simulink model "multi_model"  (R2016b)
settings: Solver=ode15s  StartTime=0.0  StopTime=inf  FixedStep=0.001  MaxStep=0.004  RelTol=1e-3
InitFcn:
  | kR_old=0;
  | kOm_old=0;
undefined symbols (not defined in the file): deg, rad, s
libraries: simulink x23, aerolibconvert2 x3, aerolibobsolete x1, aerolibtransform2 x1, aerolibatmos2 x1, aerolibnav x1, aerolibanimutils x1
(part 2 of 2)

== matlab function multi_model/control_system1/Subsystem3/Subsystem/MATLAB Function1 ==
  data: phi input; R output; theta input; psi input
function R = RPYtoRot_ZXY(phi,theta,psi)
%written by Daniel Mellinger

% BRW = [ cos(psi)*cos(theta) - sin(phi)*sin(psi)*sin(theta), 
%     cos(theta)*sin(psi) + cos(psi)*sin(phi)*sin(theta), -cos(phi)*sin(theta)]
% 
% [                                 -cos(phi)*sin(psi),
%     cos(phi)*cos(psi),             sin(phi)]
% 
% [ cos(psi)*sin(theta) + cos(theta)*sin(phi)*sin(psi), 
%     sin(psi)*sin(theta) - cos(psi)*cos(theta)*sin(phi),
%     cos(phi)*cos(theta)]

R = [ cos(psi)*cos(theta) - sin(phi)*sin(psi)*sin(theta),... 
    cos(theta)*sin(psi) + cos(psi)*sin(phi)*sin(theta), -cos(phi)*sin(theta);...
    -cos(phi)*sin(psi),...
    cos(phi)*cos(psi),             sin(phi);...
    cos(psi)*sin(theta) + cos(theta)*sin(phi)*sin(psi),...
    sin(psi)*sin(theta) - cos(psi)*cos(theta)*sin(phi),...
    cos(phi)*cos(theta)];
    
    R = R';

== matlab function multi_model/control_system1/Subsystem3/Subsystem/MATLAB Function3 ==
  data: R input; phi output; theta output; psi output
function [phi,theta,psi] = RotToRPY_ZXY(R)
%written by Daniel Mellinger

% 
% R = [ cos(psi)*cos(theta) - sin(phi)*sin(psi)*sin(theta), 
%     cos(theta)*sin(psi) + cos(psi)*sin(phi)*sin(theta), -cos(phi)*sin(theta)]
% 
% [                                 -cos(phi)*sin(psi),
%     cos(phi)*cos(psi),             sin(phi)]
% 
% [ cos(psi)*sin(theta) + cos(theta)*sin(phi)*sin(psi), 
%     sin(psi)*sin(theta) - cos(psi)*cos(theta)*sin(phi),  cos(phi)*cos(theta)]
R = R';
phi = asin(R(2,3));
psi = atan2(-R(2,1)/cos(phi),R(2,2)/cos(phi));
theta = atan2(-R(1,3)/cos(phi),R(3,3)/cos(phi));

== matlab function multi_model/control_system1/Subsystem3/Subsystem/MATLAB Function5 ==
  data: A input; t output; force input
function t = vee_map(A, force)
    if(nargin == 1)
        force = false ;
    end
    if(~force)
        if(double(sum(abs(diag(A)))) > 1e-2)
            disp('Error in vee_map() - Nonzero diagonal') ;
%             keyboard ;
        end
    end
    %A = [0 -t(3) t(2) ; t(3) 0 -t(1) ; -t(2) t(1) 0] ;
    t = [A(3,2) ;
         A(1,3) ;
         A(2,1)] ;
end

== matlab function multi_model/control_system1/pwm_out1 ==
  data: Roll input; M1 output; Pitch input; Yaw input; Thrust input; M2 output; M3 output; M4 output; M5 output; M6 output; M7 output; M8 output
function [M1, M2, M3, M4, M5, M6, M7, M8] = motor_mixer(Roll, Pitch, Yaw, Thrust)

idle_PWM = 1000;

% Quad X
M1 = ((Roll + Pitch - Yaw) / 2 * Thrust + Thrust) * 1000 + idle_PWM;
M2 = ((-Roll + Pitch + Yaw) / 2 * Thrust + Thrust) * 1000 + idle_PWM;
M3 = ((-Roll - Pitch - Yaw) / 2 * Thrust + Thrust) * 1000 + idle_PWM;
M4 = ((Roll - Pitch + Yaw) / 2 * Thrust + Thrust) * 1000 + idle_PWM;
M5 = 1000;
M6 = 1000;
M7 = 1000;
M8 = 1000;

% Quad +
% M1 = ((Pitch - Yaw) * Thrust / 2 + Thrust) * 1000 + idle_PWM;
% M2 = ((-Roll + Yaw) * Thrust / 2 + Thrust) * 1000 + idle_PWM;
% M3 = ((-Pitch - Yaw) * Thrust / 2 + Thrust) * 1000 + idle_PWM;
% M4 = ((Roll + Yaw) * Thrust / 2 + Thrust) * 1000 + idle_PWM;
% M5 = 1000;
% M6 = 1000;
% M7 = 1000;
% M8 = 1000;

% Hex X
% M1 = ((Pitch + Roll / 2 - Yaw) * Thrust / 2 + Thrust) * 1000 + idle_PWM;
% M2 = ((Pitch - Roll / 2 + Yaw) * Thrust / 2 + Thrust) * 1000 + idle_PWM;
% M3 = ((-Roll - Yaw) * Thrust / 2 + Thrust) * 1000 + idle_PWM;
% M4 = ((-Pitch - Roll / 2 + Yaw) * Thrust / 2 + Thrust) * 1000 + idle_PWM;
% M5 = ((-Pitch + Roll / 2 - Yaw) * Thrust / 2 + Thrust) * 1000 + idle_PWM;
% M6 = ((Roll + Yaw) * Thrust / 2 + Thrust) * 1000 + idle_PWM;
% M7 = 1000;
% M8 = 1000;
